simulink model "CLIK_PINV1"  (R2019b)
settings: Solver=VariableStepAuto  StartTime=0.0  StopTime=T(end)+3  RelTol=1e-3
undefined symbols (not defined in the file): a1, a2, d0, DiscIntNeverNeededParam, q0
settings Model: Creator=damia  LastModifiedBy=Alessandro
settings DataIOCC: ReturnWorkspaceOutputs=off
settings DebuggingCC: ArithmeticOperatorsInVariantConditions=warning
settings SFSimCC: CustomCodeUndefinedFunction=UseInterfaceOnly

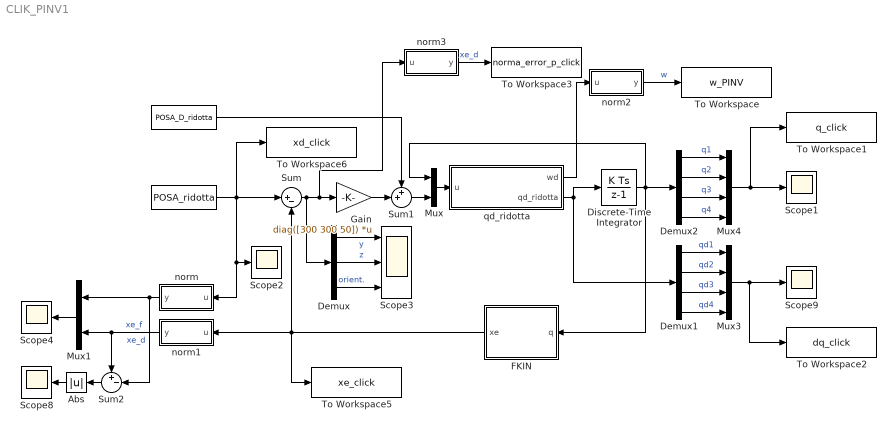
== system CLIK_PINV1 ==
  " " : FromWorkspace  VariableName=POSA_ridotta  SampleTime=0.001
  " " : FromWorkspace  VariableName=POSA_D_ridotta  SampleTime=0.001
  Abs : Abs
  Demux : Demux  Outputs=3
  Demux1 : Demux
  Demux2 : Demux
  Discrete-Time Integrator : DiscreteIntegrator  InitialCondition=q0  SampleTime=1e-3  ICPrevOutput=DiscIntNeverNeededParam  ICPrevScaledInput=DiscIntNeverNeededParam
  FKIN : MATLAB Function  TreatAsAtomicUnit=on
  Gain : Gain  Gain=diag([300 300 50])  Multiplication=Matrix(K*u)
  Mux : Mux  Inputs=2
  Mux1 : Mux  Inputs=2
  Mux3 : Mux
  Mux4 : Mux
  Scope{1..2,4,8..9} (5 alike) : Scope
  Scope3 : Scope  NumInputPorts=3
  Sum : Sum  Inputs=|+-
  Sum1 : Sum  Inputs=++|
  Sum2 : Sum  Inputs=+-|
  To Workspace : ToWorkspace  VariableName=w_PINV  SaveFormat=Timeseries  SampleTime=-1
  To Workspace1 : ToWorkspace  VariableName=q_click  SaveFormat=Timeseries  SampleTime=-1
  To Workspace2 : ToWorkspace  VariableName=dq_click  SaveFormat=Timeseries  SampleTime=-1
  To Workspace3 : ToWorkspace  VariableName=norma_error_p_click  SaveFormat=Timeseries  SampleTime=-1
  To Workspace5 : ToWorkspace  VariableName=xe_click  SaveFormat=Timeseries  SampleTime=-1
  To Workspace6 : ToWorkspace  VariableName=xd_click  SaveFormat=Timeseries  SampleTime=-1
  norm : MATLAB Function  TreatAsAtomicUnit=on
  norm1 : MATLAB Function  TreatAsAtomicUnit=on
  norm2 : MATLAB Function  TreatAsAtomicUnit=on
  norm3 : MATLAB Function  TreatAsAtomicUnit=on
  "qd_ridotta " : MATLAB Function  TreatAsAtomicUnit=on
  wires:
  " "/1 -> Sum1/1
  FKIN/1(xe) -> To Workspace5/1, norm1/1(u), Sum/2
  "qd_ridotta "/2(qd_ridotta) -> Discrete-Time Integrator/1, Demux1/1
  Mux/1 -> "qd_ridotta "/1(u)
  Gain/1 -> Sum1/2
  Sum1/1 -> Mux/2
  Discrete-Time Integrator/1 -> Demux2/1, Mux/1, FKIN/1(q)
  " "/1 -> To Workspace6/1, Sum/1, norm/1(u), Scope2/1
  Sum/1 -> Demux/1, norm3/1(u), Gain/1
  norm1/1(y) -> Sum2/1, Mux1/2  "xe_f"
  Mux1/1 -> Scope4/1
  norm/1(y) -> Mux1/1, Sum2/2  "xe_d"
  Sum2/1 -> Abs/1
  Abs/1 -> Scope8/1
  Demux/3 -> Scope3/3  "orient."
  Demux/2 -> Scope3/2  "z"
  Demux2/3 -> Mux4/3  "q3"
  Demux1/1 -> Mux3/1  "qd1"
  Demux1/2 -> Mux3/2  "qd2"
  Demux1/4 -> Mux3/4  "qd4"
  Demux1/3 -> Mux3/3  "qd3"
  Demux2/2 -> Mux4/2  "q2"
  Mux3/1 -> To Workspace2/1, Scope9/1
  Mux4/1 -> To Workspace1/1, Scope1/1
  Demux2/1 -> Mux4/1  "q1"
  Demux2/4 -> Mux4/4  "q4"
  Demux/1 -> Scope3/1  "y"
  "qd_ridotta "/1(wd) -> norm2/1(u)
  norm2/1(y) -> To Workspace/1  "w"
  norm3/1(y) -> To Workspace3/1  "xe_d"

== matlab function CLIK_PINV1/qd_ridotta  ==
  data: wd output; u input; qd_ridotta output
function [wd,qd_ridotta] = fcn(u)

a1=0.5;
a2=0.5;
q = u(1:4);
u2 = u(5:7);

q1=q(1);
q2=q(2);

% Jacobiano
J = [a1*cos(q(1))+a2*cos(q(1)+q(2))    a2*cos(q(1)+q(2))  0   0   ;
                  0                              0        1   0   ;
                  1                              1        0   1   ];


k0=10;

wd = [-(2^(1/2)*(sin(2*q1)*a1^2 + sin(2*q1 + q2)*a1*a2 + sin(2*q1 + 2*q2)*a2^2))/(2*conj((a1^2*cos(q1)^2 + a1*a2*cos(q1 + q2)*cos(q1) + a2^2*cos(q1 + q2)^2)^(1/2)));
      -(2^(1/2)*a2*sin(q1 + q2)*(2*a2*cos(q1 + q2) + a1*cos(q1)))/(2*conj((a1^2*cos(q1)^2 + a1*a2*cos(q1 + q2)*cos(q1) + a2^2*cos(q1 + q2)^2)^(1/2)));
      0;
      0];

% wd = [0; a1*a2*cos(q(2)); 0; 0];

q0d=k0*wd;
  


qd_ridotta= pinv(J)*u2+(eye(4)-pinv(J)*J)*q0d;

end

== matlab function CLIK_PINV1/FKIN ==
  data: q input; xe output; a2 parameter; a1 parameter; d0 parameter
function xe = fcn(q, a2, a1, d0)

theta1 = q(1);
theta2 = q(2);
d3 = q(3);
theta4 = q(4);

% Cinematica diretta
xe = [a1*sin(theta1)+a2*sin(theta1+theta2) ;
      d3+d0;
      theta1+theta2+theta4; ];
end

== matlab function CLIK_PINV1/norm ==
  data: u input; y output
function y = norm(u)
y = norm(u);

== matlab function CLIK_PINV1/norm1 ==
  data: u input; y output
function y = norm(u)
y = norm(u);

== matlab function CLIK_PINV1/norm2 ==
  data: u input; y output
function y = norm(u)
y = norm(u);

== matlab function CLIK_PINV1/norm3 ==
  data: u input; y output
function y = norm(u)
y = norm(u);
